simulink model "create_cycloid_vehicle_ref"  (R2024b)
settings: Solver=FixedStepAuto  StartTime=0.0  StopTime=end_time_vehicle  FixedStep=0.02  RelTol=1e-3
libraries: SignalEditorBlockLib x1
settings Model: Creator=tshintai  LastModifiedBy=tshintai
settings SolverCC: AlgebraicLoopSolver=TrustRegion
settings DataIOCC: SignalLogging=off  DSMLogging=off  SaveTime=off  ReturnWorkspaceOutputsName=turn_vehicle_ref_data
settings OptimizationCC: ReuseModelBlockBuffer=off
settings DebuggingCC: UnconnectedInputMsg=warning  UnconnectedOutputMsg=warning  UnconnectedLineMsg=warning
settings ModelReferenceCC: EnableRefExpFcnMdlSchedulingChecks=on
settings RTWCC: GPUComputeCapability=3.5  DLArmComputeVersion=19.05

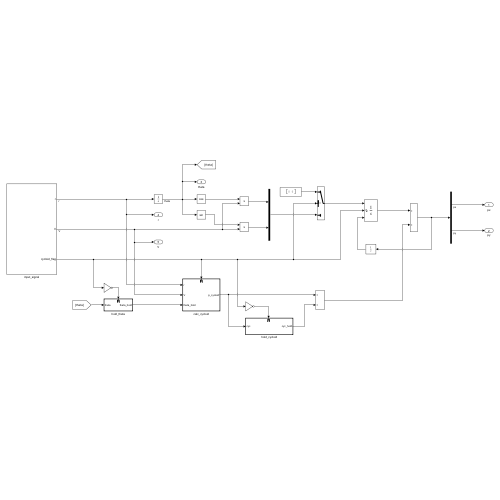
[thumbnail: Simulink's stored preview of the top-level diagram]
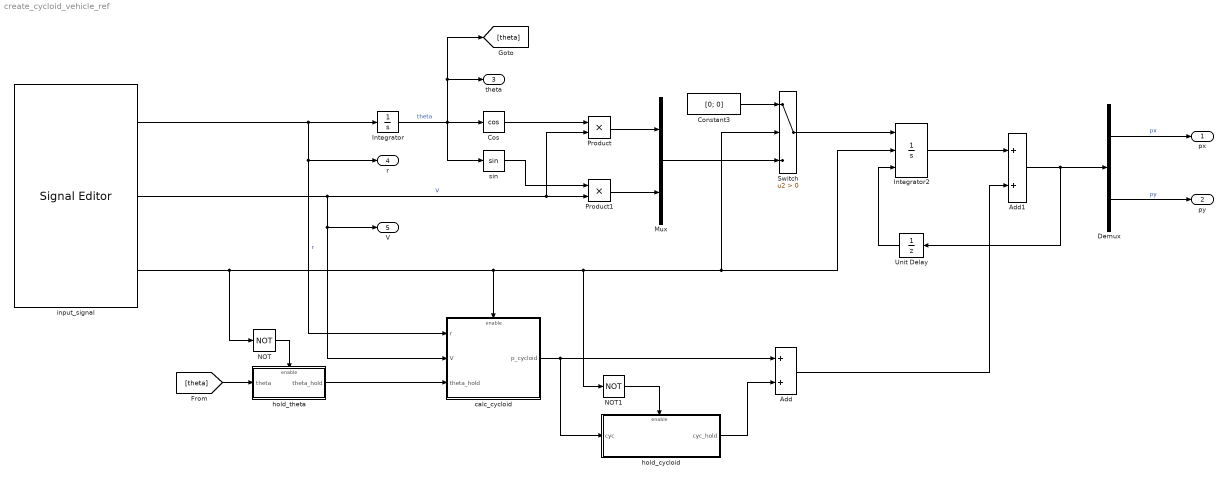
== system create_cycloid_vehicle_ref ==
  Add : Sum
  Add1 : Sum
  Constant3 : Constant  Value=[0; 0]
  Cos : Trigonometry  Operator=cos
  Demux : Demux  Outputs=2
  Integrator : Integrator
  Integrator2 : Integrator  ExternalReset=falling  InitialConditionSource=external
  Mux : Mux  Inputs=2
  NOT : Logic  Operator=NOT  IconShape=distinctive  AllPortsSameDT=off  OutDataTypeStr=boolean
  NOT1 : Logic  Operator=NOT  IconShape=distinctive  AllPortsSameDT=off  OutDataTypeStr=boolean
  Product : Product
  Product1 : Product
  Switch : Switch  Criteria=u2 > Threshold  SaturateOnIntegerOverflow=off  InputSameDT=off
  Unit Delay : UnitDelay  SampleTime=-1  HasFrameUpgradeWarning=on
  calc_cycloid : Subsystem  TreatAsAtomicUnit=on
  hold_cycloid : Subsystem  TreatAsAtomicUnit=on
  hold_theta : Subsystem  TreatAsAtomicUnit=on
  input_signal : SignalEditorBlockLib/Signal Editor  FileName=ref_elements_signal.mat  ActiveScenario=elements_of_cycloid_turn_vehicle  ActiveSignal=r  IsBus=off  OutputBusObjectStr=Bus: BusObject  SampleTime=0  ZeroCross=off  OutputAfterFinalValue=Holding final value  Unit=inherit  PreserveSignalName=on  ApplySigPropsToAllScenarios=on  ApplySigPropsToAllSignals=off
  sin : Trigonometry
  px : Outport
  py : Outport  Port=2
  theta : Outport  Port=3
  r : Outport  Port=4
  V : Outport  Port=5
  wires:
  input_signal/1 -> calc_cycloid/1(r), r/1, Integrator/1  "r"
  Integrator/1 -> [theta], theta/1, sin/1, Cos/1  "theta"
  Cos/1 -> Product/1
  input_signal/2 -> V/1, calc_cycloid/2(V), Product/2, Product1/2  "V"
  sin/1 -> Product1/1
  Product/1 -> Mux/1
  Product1/1 -> Mux/2
  Mux/1 -> Switch/3
  Demux/1 -> px/1  "px"
  Demux/2 -> py/1  "py"
  Add1/1 -> Unit Delay/1, Demux/1
  Integrator2/1 -> Add1/1
  Switch/1 -> Integrator2/1
  Constant3/1 -> Switch/1
  input_signal/3 -> NOT/1, Integrator2/2, Switch/2, NOT1/1, calc_cycloid/Enable
  [theta] -> hold_theta/1(theta)
  hold_theta/1(theta_hold) -> calc_cycloid/3(theta_hold)
  NOT/1 -> hold_theta/Enable
  calc_cycloid/1(p_cycloid) -> hold_cycloid/1(cyc), Add/1
  hold_cycloid/1(cyc_hold) -> Add/2
  NOT1/1 -> hold_cycloid/Enable
  Add/1 -> Add1/2
  Unit Delay/1 -> Integrator2/3

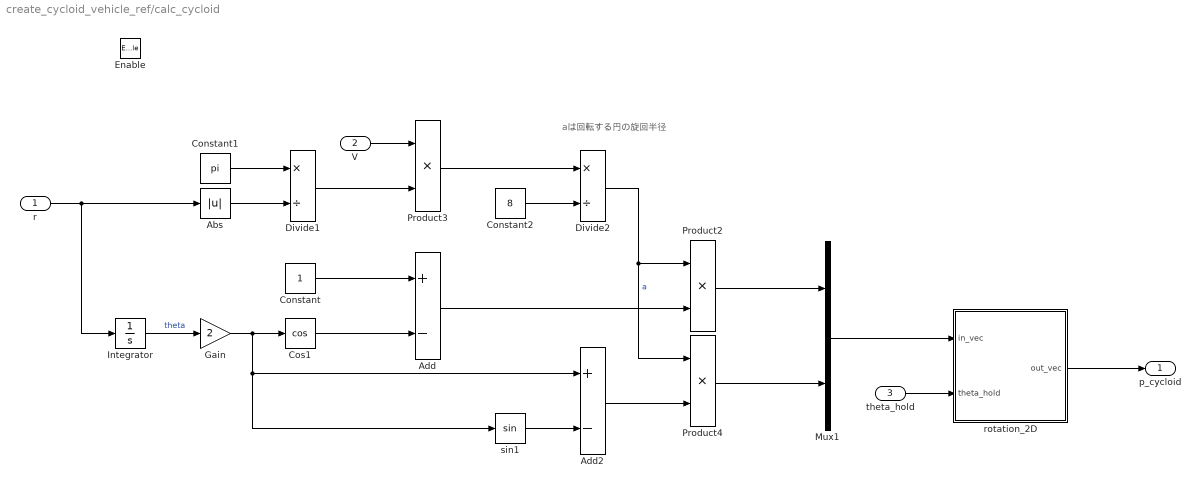
== system create_cycloid_vehicle_ref/calc_cycloid ==
  note: aは回転する円の旋回半径
  r : Inport
  V : Inport  Port=2
  theta_hold : Inport  Port=3
  Enable : EnablePort  StatesWhenEnabling=reset
  Abs : Abs  SaturateOnIntegerOverflow=off
  Add : Sum  Inputs=+-
  Add2 : Sum  Inputs=+-
  Constant : Constant
  Constant1 : Constant  Value=pi
  Constant2 : Constant  Value=8
  Cos1 : Trigonometry  Operator=cos
  Divide1 : Product  Inputs=*/
  Divide2 : Product  Inputs=*/
  Gain : Gain  Gain=2
  Integrator : Integrator
  Mux1 : Mux  Inputs=2
  Product2 : Product
  Product3 : Product
  Product4 : Product
  rotation_2D : Subsystem
  sin1 : Trigonometry
  p_cycloid : Outport  OutputWhenDisabled=reset  InitialOutput=[0; 0]
  wires:
  Cos1/1 -> Add/2
  Add2/1 -> Product4/2
  Constant2/1 -> Divide2/2
  Add/1 -> Product2/2
  Product2/1 -> Mux1/1
  Product3/1 -> Divide2/1
  Divide1/1 -> Product3/2
  Constant/1 -> Add/1
  Product4/1 -> Mux1/2
  sin1/1 -> Add2/2
  Constant1/1 -> Divide1/1
  Divide2/1 -> Product4/1, Product2/1  "a"
  V/1 -> Product3/1
  r/1 -> Integrator/1, Abs/1
  Gain/1 -> Add2/1, sin1/1, Cos1/1
  Abs/1 -> Divide1/2
  Integrator/1 -> Gain/1  "theta"
  theta_hold/1 -> rotation_2D/2(theta_hold)
  Mux1/1 -> rotation_2D/1(in_vec)
  rotation_2D/1(out_vec) -> p_cycloid/1

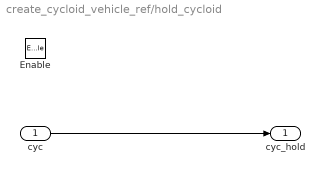
== system create_cycloid_vehicle_ref/hold_cycloid ==
  cyc : Inport
  Enable : EnablePort
  cyc_hold : Outport
  wires:
  cyc/1 -> cyc_hold/1

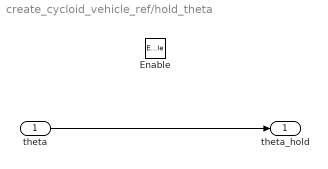
== system create_cycloid_vehicle_ref/hold_theta ==
  theta : Inport
  Enable : EnablePort
  theta_hold : Outport
  wires:
  theta/1 -> theta_hold/1

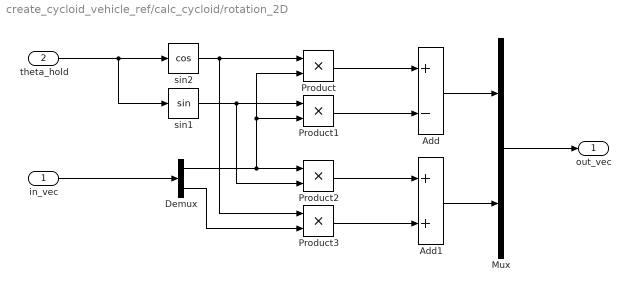
== system create_cycloid_vehicle_ref/calc_cycloid/rotation_2D ==
  in_vec : Inport
  theta_hold : Inport  Port=2
  Add : Sum  Inputs=+-
  Add1 : Sum
  Demux : Demux  Outputs=2
  Mux : Mux  Inputs=2
  Product{,1..3} (4 alike) : Product
  sin1 : Trigonometry
  sin2 : Trigonometry  Operator=cos
  out_vec : Outport
  wires:
  theta_hold/1 -> sin1/1, sin2/1
  Mux/1 -> out_vec/1
  Add/1 -> Mux/1
  Add1/1 -> Mux/2
  sin2/1 -> Product3/1, Product/1
  Product/1 -> Add/1
  Product1/1 -> Add/2
  in_vec/1 -> Demux/1
  Demux/1 -> Product2/1, Product1/2, Product/2
  sin1/1 -> Product2/2, Product1/1
  Product3/1 -> Add1/2
  Product2/1 -> Add1/1
  Demux/2 -> Product3/2
